simulink model "LQG_no_integrator"  (R2022b)
settings: Solver=VariableStepAuto  StartTime=0.0  StopTime=200  RelTol=1e-3
values from neighbouring files (symbols this model uses):
  J = get_linearization()    [LQG.m]
  Kr = lqr(A,B,Q,R)    [LQG.m]
undefined symbols (not defined in the file or in its folder): Ke, std_dev_dy, std_dev_phi_dot, std_dev_psi, std_dev_tau_phi, std_dev_theta, X_start
libraries: simulink x2
settings Model: Creator=alexi  LastModifiedBy=franc

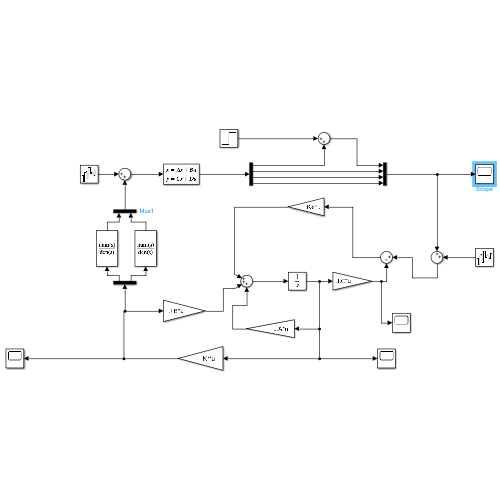
[thumbnail: Simulink's stored preview of the top-level diagram]
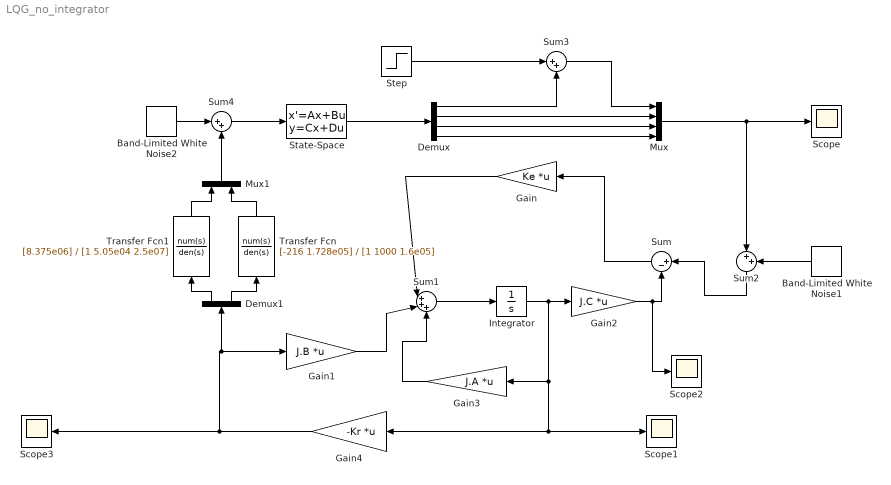
== system LQG_no_integrator ==
  Band-Limited White Noise1 : simulink/Sources/Band-Limited White Noise  Cov=[std_dev_dy^2; std_dev_theta^2; std_dev_phi_dot^2; std_dev_psi^2]  Ts=0.1  seed=[23341]
  Band-Limited White Noise2 : simulink/Sources/Band-Limited White Noise  Cov=[std_dev_tau_phi^2; std_dev_psi^2]  Ts=0.1  seed=[23341]
  Demux : Demux
  Demux1 : Demux  Outputs=2
  Gain : Gain  Gain=Ke  Multiplication=Matrix(K*u)
  Gain1 : Gain  Gain=J.B  Multiplication=Matrix(K*u)
  Gain2 : Gain  Gain=J.C  Multiplication=Matrix(K*u)
  Gain3 : Gain  Gain=J.A  Multiplication=Matrix(K*u)
  Gain4 : Gain  Gain=-Kr  Multiplication=Matrix(K*u)
  Integrator : Integrator
  Mux : Mux
  Mux1 : Mux  Inputs=2
  Scope{,1..3} (4 alike) : Scope
  State-Space : StateSpace  A=J.A  B=J.B  C=J.C  D=J.D  InitialCondition=X_start
  Step : Step  SampleTime=0
  Sum : Sum  Inputs=|+-
  Sum1 : Sum  Inputs=|+++
  Sum2 : Sum  Inputs=|++
  Sum3 : Sum  Inputs=|++
  Sum4 : Sum  Inputs=|++
  Transfer Fcn : TransferFcn  Numerator=[-216 1.728e05]  Denominator=[1 1000 1.6e05]
  Transfer Fcn1 : TransferFcn  Numerator=[8.375e06]  Denominator=[1 5.05e04 2.5e07]
  wires:
  Gain4/1 -> Gain1/1, Demux1/1, Scope3/1
  Gain/1 -> Sum1/1
  Gain1/1 -> Sum1/2
  Sum1/1 -> Integrator/1
  Integrator/1 -> Scope1/1, Gain4/1, Gain3/1, Gain2/1
  Gain2/1 -> Scope2/1, Sum/2
  Gain3/1 -> Sum1/3
  Sum2/1 -> Sum/1
  Sum/1 -> Gain/1
  State-Space/1 -> Demux/1
  Demux/1 -> Sum3/2
  Sum3/1 -> Mux/1
  Demux/2 -> Mux/2
  Demux/3 -> Mux/3
  Demux/4 -> Mux/4
  Mux/1 -> Scope/1, Sum2/1
  Band-Limited White Noise1/1 -> Sum2/2
  Step/1 -> Sum3/1
  Sum4/1 -> State-Space/1
  Band-Limited White Noise2/1 -> Sum4/1
  Demux1/2 -> Transfer Fcn/1
  Demux1/1 -> Transfer Fcn1/1
  Transfer Fcn1/1 -> Mux1/1
  Transfer Fcn/1 -> Mux1/2
  Mux1/1 -> Sum4/2
